simulink model "economy_sim"  (R2020a)
settings: Solver=VariableStepAuto  StartTime=0.0  StopTime=10.0  RelTol=1e-3
values from neighbouring files (symbols this model uses):
  start_f = temp    (= 1)    [bank_and_economy.m]    (also in economy.m = 100)
  start_g = temp    (= 1)    [bank_and_economy.m]    (also in economy.m = 100)
  start_h = temp    (= 1)    [bank_and_economy.m]    (also in economy.m = 100)
  T_f = 0.5    [a_1.m]    (also in a_2.m; a_loss_function.m; bank_and_economy.m; bank_centralbank.m)
  T_g = 1    [a_1.m]    (also in a_2.m; a_loss_function.m; bank_and_economy.m; bank_centralbank.m)
  T_h = 0.1    [a_1.m]    (also in a_2.m; a_loss_function.m; bank_and_economy.m; bank_centralbank.m)
  T_k = 0.1    [a_1.m]    (also in a_2.m; a_loss_function.m; bank_and_economy.m = 0.25; economy.m = 1)
  tx = 0.3    [a_1.m]    (also in a_2.m; a_loss_function.m; bank_and_economy.m = 0.5; bank_centralbank.m = 0.25)
settings Model: Creator=erlended  LastModifiedBy=erlended

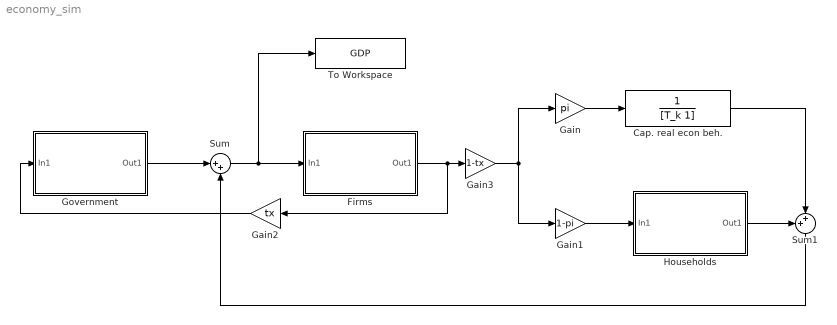
== system economy_sim ==
  Cap. real econ beh. : TransferFcn  Denominator=[T_k 1]
  Firms : Subsystem
  Gain : Gain  Gain=pi
  Gain1 : Gain  Gain=1-pi
  Gain2 : Gain  Gain=tx
  Gain3 : Gain  Gain=1-tx
  Government : Subsystem
  Households : Subsystem
  Sum : Sum  Inputs=|++
  Sum1 : Sum  Inputs=++|
  To Workspace : ToWorkspace  VariableName=GDP  SaveFormat=Timeseries  SampleTime=-1
  wires:
  Firms/1(Out1) -> Gain3/1, Gain2/1
  Gain/1 -> Cap. real econ beh./1
  Gain1/1 -> Households/1(In1)
  Sum/1 -> Firms/1(In1), To Workspace/1
  Gain3/1 -> Gain/1, Gain1/1
  Cap. real econ beh./1 -> Sum1/2
  Households/1(Out1) -> Sum1/1
  Sum1/1 -> Sum/2
  Gain2/1 -> Government/1(In1)
  Government/1(Out1) -> Sum/1

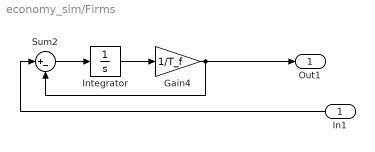
== system economy_sim/Firms ==
  In1 : Inport
  Gain4 : Gain  Gain=1/T_f
  Integrator : Integrator  InitialCondition=start_f
  Sum2 : Sum  Inputs=|+-
  Out1 : Outport
  wires:
  In1/1 -> Sum2/1
  Sum2/1 -> Integrator/1
  Gain4/1 -> Out1/1, Sum2/2
  Integrator/1 -> Gain4/1

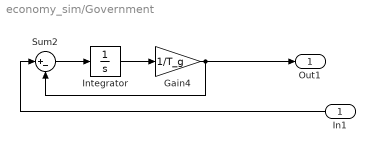
== system economy_sim/Government ==
  In1 : Inport
  Gain4 : Gain  Gain=1/T_g
  Integrator : Integrator  InitialCondition=start_g
  Sum2 : Sum  Inputs=|+-
  Out1 : Outport
  wires:
  In1/1 -> Sum2/1
  Sum2/1 -> Integrator/1
  Gain4/1 -> Out1/1, Sum2/2
  Integrator/1 -> Gain4/1

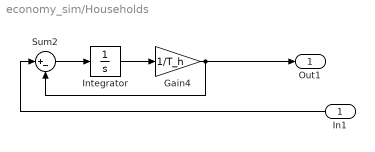
== system economy_sim/Households ==
  In1 : Inport
  Gain4 : Gain  Gain=1/T_h
  Integrator : Integrator  InitialCondition=start_h
  Sum2 : Sum  Inputs=|+-
  Out1 : Outport
  wires:
  In1/1 -> Sum2/1
  Sum2/1 -> Integrator/1
  Gain4/1 -> Out1/1, Sum2/2
  Integrator/1 -> Gain4/1
